simulink model "UAV_Task3"  (R2024b)
settings: Solver=VariableStepAuto  StartTime=0  StopTime=200  RelTol=1e-5  AbsTol=1e-5
values from neighbouring files (symbols this model uses):
  adaptiveActivation = 1    [Simplified_UAV_Task3_main.m]    (also in newUAV_Task3_main.m)
  B_p = 1/UAV.m    [Simplified_UAV_Task3_main.m]    (also in newUAV_Task3_main.m)
  F2plus = F2'*pinv(F2*F2')    [Simplified_UAV_Task3_main.m]    (also in newUAV_Task3_main.m)
  Gamma_a = 1*[1 1 1 1]'    [Simplified_UAV_Task3_main.m]    (also in newUAV_Task3_main.m = 2*[1 1 1 1]')
  gravityInAdaptiveController = 1    [Simplified_UAV_Task3_main.m]    (also in newUAV_Task3_main.m)
  k_f = 0.3379e-6    (= 3.379e-07)    [Simplified_UAV_Task3_main.m]    (also in newUAV_Task3_main.m)
  L = 10    [Simplified_UAV_Task3_main.m]    (also in newUAV_Task3_main.m)
  lambda_0 = 1    [Simplified_UAV_Task3_main.m]    (also in newUAV_Task3_main.m)
  Omega_0 = [1500 1500 1500 1500]'    [Simplified_UAV_Task3_main.m]    (also in newUAV_Task3_main.m)
  omegab_0 = [0; 0; 0]    [Simplified_UAV_Task3_main.m]    (also in newUAV_Task3_main.m)
  p_0 = [0; 0; 0]    [Simplified_UAV_Task3_main.m]    (also in newUAV_Task3_main.m)
  PO = 1    [Simplified_UAV_Task3_main.m]    (also in newUAV_Task3_main.m)
  q_0 = eul2quat([0, 0, 0]*degToRad,'ZYX')'    [Simplified_UAV_Task3_main.m]    (also in newUAV_Task3_main.m)
  scenario = 2    [Simplified_UAV_Task3_main.m]    (also in newUAV_Task3_main.m)
  theta_0 = [0.07;0.07;0.1]    [Simplified_UAV_Task3_main.m]    (also in newUAV_Task3_main.m)
  vb_0 = [0; 0; 0]    [Simplified_UAV_Task3_main.m]    (also in newUAV_Task3_main.m)
undefined symbols (not defined in the file or in its folder): adaptive_controller, ctrl, D_fv_i, dyn, e_3, epsilon_PO, fw_params_fc, g, Gamma_a_scalar, lambda_i, par, pos, pos_pp, projection_operator, targetParams, theta_M, UAV, v_M, vel, vel_pp
libraries: slpidlib x22, matrix_library x6, aerolibutil x2, uavutilslib x1
(part 2 of 4)

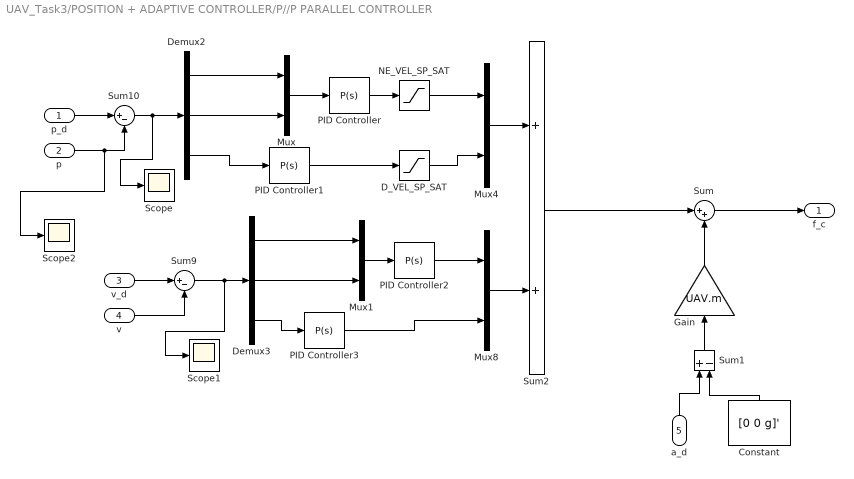
== system UAV_Task3/POSITION + ADAPTIVE CONTROLLER/P//P PARALLEL CONTROLLER ==
  p_d : Inport
  p : Inport  Port=2
  v_d : Inport  Port=3
  v : Inport  Port=4
  a_d : Inport  Port=5
  Constant : Constant  Value=[0 0 g]'
  D_VEL_SP_SAT : Saturate  UpperLimit=fw_params_fc.MPC_Z_VEL_MAX_DN  LowerLimit=-fw_params_fc.MPC_Z_VEL_MAX_UP
  Demux2 : Demux  Outputs=3
  Demux3 : Demux  Outputs=3
  Gain : Gain  Gain=UAV.m
  Mux{,1,4,8} (4 alike) : Mux  Inputs=2
  NE_VEL_SP_SAT : Saturate  UpperLimit=fw_params_fc.MPC_XY_VEL_MAX  LowerLimit=-fw_params_fc.MPC_XY_VEL_MAX
  PID Controller : slpidlib/PID Controller  Controller=P  Form=Parallel  TimeDomain=Continuous-time  UseExternalTs=off  SampleTime=-1  IntegratorMethod=Forward Euler  FilterMethod=Forward Euler  ControllerParametersSource=internal  P=pos_pp.Kp(1,1)  I=1  UseKiTs=off  D=0  UseExternalDerivativeSource=off  N=100  UseFilter=on  TunerSelectOption=Transfer Function Based (PID Tuner App)  InitialConditionSource=internal  InitialConditionForIntegrator=0  InitialConditionForFilter=0  DifferentiatorICPrevScaledInput=0  ExternalReset=none  TrackingMode=off  Kt=1  LimitOutput=off  SatLimitsSource=internal  UpperSaturationLimit=inf  LowerSaturationLimit=-inf  LinearizeAsGain=on  AntiWindupMode=none  Kb=1  LimitIntegrator=off  UpperIntegratorSaturationLimit=inf  LowerIntegratorSaturationLimit=-inf  POutMin=[]  POutMax=[]  IOutMin=[]  IOutMax=[]  DOutMin=[]  DOutMax=[]  NOutMin=[]  NOutMax=[]  SumOutMin=[]  SumOutMax=[]  SaturationOutMin=[]  SaturationOutMax=[]  PParamMin=[]  PParamMax=[]  IParamMin=[]  IParamMax=[]  DParamMin=[]  DParamMax=[]  NParamMin=[]  NParamMax=[]  KbParamMin=[]  KbParamMax=[]  KtParamMin=[]  KtParamMax=[]  KbOutMin=[]  KbOutMax=[]  KtOutMin=[]  KtOutMax=[]  IntegratorOutMin=[]  IntegratorOutMax=[]  FilterOutMin=[]  FilterOutMax=[]  SumI1OutMin=[]  SumI1OutMax=[]  SumI2OutMin=[]  SumI2OutMax=[]  SumI3OutMin=[]  SumI3OutMax=[]  SumI4OutMin=[]  SumI4OutMax=[]  SumDOutMin=[]  SumDOutMax=[]  DifferentiatorOutMin=[]  DifferentiatorOutMax=[]  FilterDiffOutCoefMin=[]  FilterDiffOutCoefMax=[]  ReciprocalOutMin=[]  ReciprocalOutMax=[]  SumDenOutMin=[]  SumDenOutMax=[]  SumNumOutMin=[]  SumNumOutMax=[]  DivideOutMin=[]  DivideOutMax=[]  UdiffTsProdOutMin=[]  UdiffTsProdOutMax=[]  NTsProdOutMin=[]  NTsProdOutMax=[]  UintegralTsProdOutMin=[]  UintegralTsProdOutMax=[]  UngainTsProdOutMin=[]  UngainTsProdOutMax=[]  ClampingZeroOutDataTypeStr=Inherit: Inherit via back propagation  ClampingZeroOutMin=[]  ClampingZeroOutMax=[]  FilterDenConstantOutDataTypeStr=Inherit: Inherit via back propagation  FilterDenConstantOutMin=[]  FilterDenConstantOutMax=[]  PCopyOutDataTypeStr=Inherit: Inherit via back propagation  PCopyOutMin=[]  PCopyOutMax=[]  NCopyOutDataTypeStr=Inherit: Inherit via back propagation  NCopyOutMin=[]  NCopyOutMax=[]  IntegratorContinuousStateAttributes=''  IntegratorStateMustResolveToSignalObject=off  IntegratorRTWStateStorageClass=Auto  FilterContinuousStateAttributes=''  FilterStateMustResolveToSignalObject=off  FilterRTWStateStorageClass=Auto  ParallelPVariant=InternalParameters  IdealPVariant=Disabled  IVariant=Disabled  DVariant=Disabled  IntegratorVariant=Disabled  SatVariant=Disabled  AWVariant=Disabled  PCopyVariant=Disabled  TRVariant=Disabled  FdbkBlocksVariant=Forward  IdealPFdbkVariant=Disabled  SatFdbkVariant=Disabled  DerivativeFilterVariant=Disabled  NVariant=Disabled  NCopyVariant=Disabled_SignalSpec  FilterICVariant=Disabled  IntegratorICVariant=Disabled  ExternalResetVariant=Disabled  TRSumVariant=Passthrough  SumFdbkVariant=Disabled  SumVariant=Passthrough_P  TsampFilterVariant=InternalTs  TsampNgainVariant=Passthrough  TsampIntegralVariant=Disabled_SignalSpec  ExternalSaturationOutDataTypeStr=Inherit: Same as second input  DerivativeSourceVariant=Disabled  PreIntVariant=InternalPreInt
  PID Controller1 : slpidlib/PID Controller  Controller=P  Form=Parallel  TimeDomain=Continuous-time  UseExternalTs=off  SampleTime=-1  IntegratorMethod=Forward Euler  FilterMethod=Forward Euler  ControllerParametersSource=internal  P=pos_pp.Kp(3,3)  I=6.65250446585681  UseKiTs=off  D=9.35493624576525  UseExternalDerivativeSource=off  N=3445.77467620609  UseFilter=on  TunerSelectOption=Transfer Function Based (PID Tuner App)  InitialConditionSource=internal  InitialConditionForIntegrator=0  InitialConditionForFilter=0  DifferentiatorICPrevScaledInput=0  ExternalReset=none  TrackingMode=off  Kt=1  LimitOutput=off  SatLimitsSource=internal  UpperSaturationLimit=inf  LowerSaturationLimit=-inf  LinearizeAsGain=on  AntiWindupMode=none  Kb=1  LimitIntegrator=off  UpperIntegratorSaturationLimit=inf  LowerIntegratorSaturationLimit=-inf  POutMin=[]  POutMax=[]  IOutMin=[]  IOutMax=[]  DOutMin=[]  DOutMax=[]  NOutMin=[]  NOutMax=[]  SumOutMin=[]  SumOutMax=[]  SaturationOutMin=[]  SaturationOutMax=[]  PParamMin=[]  PParamMax=[]  IParamMin=[]  IParamMax=[]  DParamMin=[]  DParamMax=[]  NParamMin=[]  NParamMax=[]  KbParamMin=[]  KbParamMax=[]  KtParamMin=[]  KtParamMax=[]  KbOutMin=[]  KbOutMax=[]  KtOutMin=[]  KtOutMax=[]  IntegratorOutMin=[]  IntegratorOutMax=[]  FilterOutMin=[]  FilterOutMax=[]  SumI1OutMin=[]  SumI1OutMax=[]  SumI2OutMin=[]  SumI2OutMax=[]  SumI3OutMin=[]  SumI3OutMax=[]  SumI4OutMin=[]  SumI4OutMax=[]  SumDOutMin=[]  SumDOutMax=[]  DifferentiatorOutMin=[]  DifferentiatorOutMax=[]  FilterDiffOutCoefMin=[]  FilterDiffOutCoefMax=[]  ReciprocalOutMin=[]  ReciprocalOutMax=[]  SumDenOutMin=[]  SumDenOutMax=[]  SumNumOutMin=[]  SumNumOutMax=[]  DivideOutMin=[]  DivideOutMax=[]  UdiffTsProdOutMin=[]  UdiffTsProdOutMax=[]  NTsProdOutMin=[]  NTsProdOutMax=[]  UintegralTsProdOutMin=[]  UintegralTsProdOutMax=[]  UngainTsProdOutMin=[]  UngainTsProdOutMax=[]  ClampingZeroOutDataTypeStr=Inherit: Inherit via back propagation  ClampingZeroOutMin=[]  ClampingZeroOutMax=[]  FilterDenConstantOutDataTypeStr=Inherit: Inherit via back propagation  FilterDenConstantOutMin=[]  FilterDenConstantOutMax=[]  PCopyOutDataTypeStr=Inherit: Inherit via back propagation  PCopyOutMin=[]  PCopyOutMax=[]  NCopyOutDataTypeStr=Inherit: Inherit via back propagation  NCopyOutMin=[]  NCopyOutMax=[]  IntegratorContinuousStateAttributes=''  IntegratorStateMustResolveToSignalObject=off  IntegratorRTWStateStorageClass=Auto  FilterContinuousStateAttributes=''  FilterStateMustResolveToSignalObject=off  FilterRTWStateStorageClass=Auto  ParallelPVariant=InternalParameters  IdealPVariant=Disabled  IVariant=Disabled  DVariant=Disabled  IntegratorVariant=Disabled  SatVariant=Disabled  AWVariant=Disabled  PCopyVariant=Disabled  TRVariant=Disabled  FdbkBlocksVariant=Forward  IdealPFdbkVariant=Disabled  SatFdbkVariant=Disabled  DerivativeFilterVariant=Disabled  NVariant=Disabled  NCopyVariant=Disabled_SignalSpec  FilterICVariant=Disabled  IntegratorICVariant=Disabled  ExternalResetVariant=Disabled  TRSumVariant=Passthrough  SumFdbkVariant=Disabled  SumVariant=Passthrough_P  TsampFilterVariant=InternalTs  TsampNgainVariant=Passthrough  TsampIntegralVariant=Disabled_SignalSpec  ExternalSaturationOutDataTypeStr=Inherit: Same as second input  DerivativeSourceVariant=Disabled  PreIntVariant=InternalPreInt
  PID Controller2 : slpidlib/PID Controller  Controller=P  Form=Parallel  TimeDomain=Continuous-time  UseExternalTs=off  SampleTime=-1  IntegratorMethod=Forward Euler  FilterMethod=Forward Euler  ControllerParametersSource=internal  P=vel_pp.Kp(1,1)  I=1  UseKiTs=off  D=0  UseExternalDerivativeSource=off  N=100  UseFilter=on  TunerSelectOption=Transfer Function Based (PID Tuner App)  InitialConditionSource=internal  InitialConditionForIntegrator=0  InitialConditionForFilter=0  DifferentiatorICPrevScaledInput=0  ExternalReset=none  TrackingMode=off  Kt=1  LimitOutput=off  SatLimitsSource=internal  UpperSaturationLimit=inf  LowerSaturationLimit=-inf  LinearizeAsGain=on  AntiWindupMode=none  Kb=1  LimitIntegrator=off  UpperIntegratorSaturationLimit=inf  LowerIntegratorSaturationLimit=-inf  POutMin=[]  POutMax=[]  IOutMin=[]  IOutMax=[]  DOutMin=[]  DOutMax=[]  NOutMin=[]  NOutMax=[]  SumOutMin=[]  SumOutMax=[]  SaturationOutMin=[]  SaturationOutMax=[]  PParamMin=[]  PParamMax=[]  IParamMin=[]  IParamMax=[]  DParamMin=[]  DParamMax=[]  NParamMin=[]  NParamMax=[]  KbParamMin=[]  KbParamMax=[]  KtParamMin=[]  KtParamMax=[]  KbOutMin=[]  KbOutMax=[]  KtOutMin=[]  KtOutMax=[]  IntegratorOutMin=[]  IntegratorOutMax=[]  FilterOutMin=[]  FilterOutMax=[]  SumI1OutMin=[]  SumI1OutMax=[]  SumI2OutMin=[]  SumI2OutMax=[]  SumI3OutMin=[]  SumI3OutMax=[]  SumI4OutMin=[]  SumI4OutMax=[]  SumDOutMin=[]  SumDOutMax=[]  DifferentiatorOutMin=[]  DifferentiatorOutMax=[]  FilterDiffOutCoefMin=[]  FilterDiffOutCoefMax=[]  ReciprocalOutMin=[]  ReciprocalOutMax=[]  SumDenOutMin=[]  SumDenOutMax=[]  SumNumOutMin=[]  SumNumOutMax=[]  DivideOutMin=[]  DivideOutMax=[]  UdiffTsProdOutMin=[]  UdiffTsProdOutMax=[]  NTsProdOutMin=[]  NTsProdOutMax=[]  UintegralTsProdOutMin=[]  UintegralTsProdOutMax=[]  UngainTsProdOutMin=[]  UngainTsProdOutMax=[]  ClampingZeroOutDataTypeStr=Inherit: Inherit via back propagation  ClampingZeroOutMin=[]  ClampingZeroOutMax=[]  FilterDenConstantOutDataTypeStr=Inherit: Inherit via back propagation  FilterDenConstantOutMin=[]  FilterDenConstantOutMax=[]  PCopyOutDataTypeStr=Inherit: Inherit via back propagation  PCopyOutMin=[]  PCopyOutMax=[]  NCopyOutDataTypeStr=Inherit: Inherit via back propagation  NCopyOutMin=[]  NCopyOutMax=[]  IntegratorContinuousStateAttributes=''  IntegratorStateMustResolveToSignalObject=off  IntegratorRTWStateStorageClass=Auto  FilterContinuousStateAttributes=''  FilterStateMustResolveToSignalObject=off  FilterRTWStateStorageClass=Auto  ParallelPVariant=InternalParameters  IdealPVariant=Disabled  IVariant=Disabled  DVariant=Disabled  IntegratorVariant=Disabled  SatVariant=Disabled  AWVariant=Disabled  PCopyVariant=Disabled  TRVariant=Disabled  FdbkBlocksVariant=Forward  IdealPFdbkVariant=Disabled  SatFdbkVariant=Disabled  DerivativeFilterVariant=Disabled  NVariant=Disabled  NCopyVariant=Disabled_SignalSpec  FilterICVariant=Disabled  IntegratorICVariant=Disabled  ExternalResetVariant=Disabled  TRSumVariant=Passthrough  SumFdbkVariant=Disabled  SumVariant=Passthrough_P  TsampFilterVariant=InternalTs  TsampNgainVariant=Passthrough  TsampIntegralVariant=Disabled_SignalSpec  ExternalSaturationOutDataTypeStr=Inherit: Same as second input  DerivativeSourceVariant=Disabled  PreIntVariant=InternalPreInt
  PID Controller3 : slpidlib/PID Controller  Controller=P  Form=Parallel  TimeDomain=Continuous-time  UseExternalTs=off  SampleTime=-1  IntegratorMethod=Forward Euler  FilterMethod=Forward Euler  ControllerParametersSource=internal  P=vel_pp.Kp(3,3)  I=1  UseKiTs=off  D=0  UseExternalDerivativeSource=off  N=100  UseFilter=on  TunerSelectOption=Transfer Function Based (PID Tuner App)  InitialConditionSource=internal  InitialConditionForIntegrator=0  InitialConditionForFilter=0  DifferentiatorICPrevScaledInput=0  ExternalReset=none  TrackingMode=off  Kt=1  LimitOutput=off  SatLimitsSource=internal  UpperSaturationLimit=inf  LowerSaturationLimit=-inf  LinearizeAsGain=on  AntiWindupMode=none  Kb=1  LimitIntegrator=off  UpperIntegratorSaturationLimit=inf  LowerIntegratorSaturationLimit=-inf  POutMin=[]  POutMax=[]  IOutMin=[]  IOutMax=[]  DOutMin=[]  DOutMax=[]  NOutMin=[]  NOutMax=[]  SumOutMin=[]  SumOutMax=[]  SaturationOutMin=[]  SaturationOutMax=[]  PParamMin=[]  PParamMax=[]  IParamMin=[]  IParamMax=[]  DParamMin=[]  DParamMax=[]  NParamMin=[]  NParamMax=[]  KbParamMin=[]  KbParamMax=[]  KtParamMin=[]  KtParamMax=[]  KbOutMin=[]  KbOutMax=[]  KtOutMin=[]  KtOutMax=[]  IntegratorOutMin=[]  IntegratorOutMax=[]  FilterOutMin=[]  FilterOutMax=[]  SumI1OutMin=[]  SumI1OutMax=[]  SumI2OutMin=[]  SumI2OutMax=[]  SumI3OutMin=[]  SumI3OutMax=[]  SumI4OutMin=[]  SumI4OutMax=[]  SumDOutMin=[]  SumDOutMax=[]  DifferentiatorOutMin=[]  DifferentiatorOutMax=[]  FilterDiffOutCoefMin=[]  FilterDiffOutCoefMax=[]  ReciprocalOutMin=[]  ReciprocalOutMax=[]  SumDenOutMin=[]  SumDenOutMax=[]  SumNumOutMin=[]  SumNumOutMax=[]  DivideOutMin=[]  DivideOutMax=[]  UdiffTsProdOutMin=[]  UdiffTsProdOutMax=[]  NTsProdOutMin=[]  NTsProdOutMax=[]  UintegralTsProdOutMin=[]  UintegralTsProdOutMax=[]  UngainTsProdOutMin=[]  UngainTsProdOutMax=[]  ClampingZeroOutDataTypeStr=Inherit: Inherit via back propagation  ClampingZeroOutMin=[]  ClampingZeroOutMax=[]  FilterDenConstantOutDataTypeStr=Inherit: Inherit via back propagation  FilterDenConstantOutMin=[]  FilterDenConstantOutMax=[]  PCopyOutDataTypeStr=Inherit: Inherit via back propagation  PCopyOutMin=[]  PCopyOutMax=[]  NCopyOutDataTypeStr=Inherit: Inherit via back propagation  NCopyOutMin=[]  NCopyOutMax=[]  IntegratorContinuousStateAttributes=''  IntegratorStateMustResolveToSignalObject=off  IntegratorRTWStateStorageClass=Auto  FilterContinuousStateAttributes=''  FilterStateMustResolveToSignalObject=off  FilterRTWStateStorageClass=Auto  ParallelPVariant=InternalParameters  IdealPVariant=Disabled  IVariant=Disabled  DVariant=Disabled  IntegratorVariant=Disabled  SatVariant=Disabled  AWVariant=Disabled  PCopyVariant=Disabled  TRVariant=Disabled  FdbkBlocksVariant=Forward  IdealPFdbkVariant=Disabled  SatFdbkVariant=Disabled  DerivativeFilterVariant=Disabled  NVariant=Disabled  NCopyVariant=Disabled_SignalSpec  FilterICVariant=Disabled  IntegratorICVariant=Disabled  ExternalResetVariant=Disabled  TRSumVariant=Passthrough  SumFdbkVariant=Disabled  SumVariant=Passthrough_P  TsampFilterVariant=InternalTs  TsampNgainVariant=Passthrough  TsampIntegralVariant=Disabled_SignalSpec  ExternalSaturationOutDataTypeStr=Inherit: Same as second input  DerivativeSourceVariant=Disabled  PreIntVariant=InternalPreInt
  Scope : Scope
  Scope1 : Scope
  Scope2 : Scope
  Sum : Sum  Inputs=|++
  Sum1 : Sum  Inputs=+-
  Sum10 : Sum  Inputs=|+-
  Sum2 : Sum
  Sum9 : Sum  Inputs=|+-
  f_c : Outport
  wires:
  p_d/1 -> Sum10/1
  p/1 -> Scope2/1, Sum10/2
  v_d/1 -> Sum9/1
  Sum9/1 -> Scope1/1, Demux3/1
  Sum10/1 -> Scope/1, Demux2/1
  Demux3/3 -> PID Controller3/1
  v/1 -> Sum9/2
  Demux2/3 -> PID Controller1/1
  Mux4/1 -> Sum2/1
  Mux8/1 -> Sum2/2
  Demux2/2 -> Mux/2
  Sum/1 -> f_c/1
  Gain/1 -> Sum/2
  Sum1/1 -> Gain/1
  a_d/1 -> Sum1/1
  Constant/1 -> Sum1/2
  Sum2/1 -> Sum/1
  Mux/1 -> PID Controller/1
  Demux2/1 -> Mux/1
  Demux3/1 -> Mux1/1
  Demux3/2 -> Mux1/2
  Mux1/1 -> PID Controller2/1
  PID Controller3/1 -> Mux8/2
  PID Controller2/1 -> Mux8/1
  PID Controller/1 -> NE_VEL_SP_SAT/1
  NE_VEL_SP_SAT/1 -> Mux4/1
  PID Controller1/1 -> D_VEL_SP_SAT/1
  D_VEL_SP_SAT/1 -> Mux4/2

== system UAV_Task3/POSITION + ADAPTIVE CONTROLLER/POSITION CONTROLLER ==
  p_d : Inport
  p : Inport  Port=2
  v_d : Inport  Port=3
  v : Inport  Port=4
  a_d : Inport  Port=5
  Position controller : Subsystem
  Scope : Scope
  Sum : Sum  Inputs=|+-
  Velocity Controller : Subsystem
  f_c : Outport
  wires:
  v/1 -> Position controller/5(v), Velocity Controller/1(v)
  Position controller/1(" v_c") -> Velocity Controller/2(v_c)
  Position controller/2(" a_c") -> Velocity Controller/3(a_c)
  a_d/1 -> Position controller/4(a_d)
  v_d/1 -> Position controller/3(v_d)
  p/1 -> Sum/1, Position controller/1(p)
  p_d/1 -> Sum/2, Position controller/2(p_d)
  Sum/1 -> Scope/1
  Velocity Controller/1(f_c) -> f_c/1

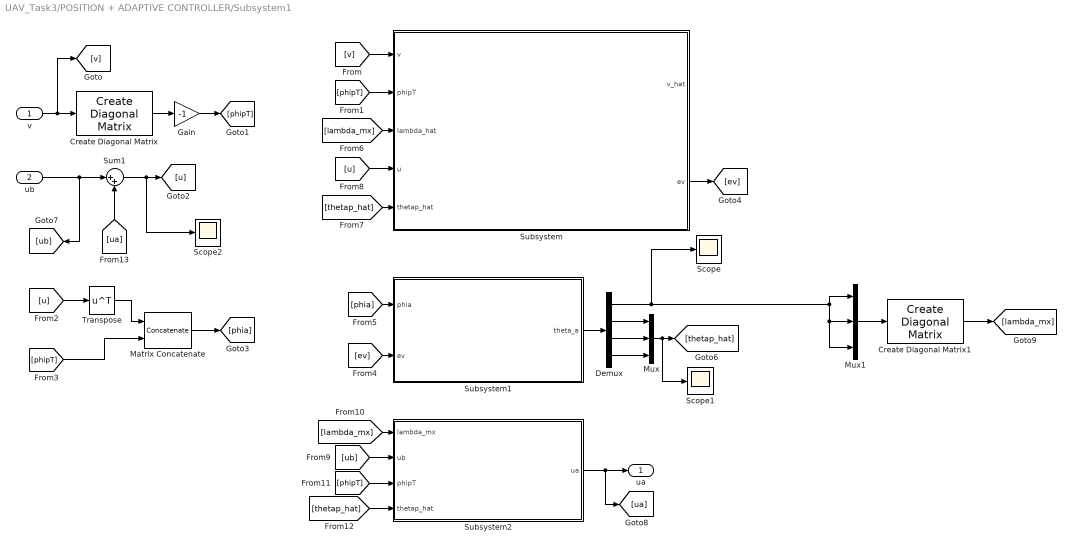
== system UAV_Task3/POSITION + ADAPTIVE CONTROLLER/Subsystem1 ==
  v : Inport
  ub : Inport  Port=2
  Create Diagonal Matrix : matrix_library/Create Diagonal Matrix
  Create Diagonal Matrix1 : matrix_library/Create Diagonal Matrix
  Demux : Demux
  Gain : Gain  Gain=-1
  Matrix Concatenate : Concatenate  Mode=Multidimensional array
  Mux : Mux  Inputs=3
  Mux1 : Mux  Inputs=3
  Scope : Scope
  Scope1 : Scope
  Scope2 : Scope
  Subsystem : Subsystem
  Subsystem1 : Subsystem
  Subsystem2 : Subsystem
  Sum1 : Sum  Inputs=|++
  Transpose : Math  Operator=transpose
  ua : Outport
  wires:
  v/1 -> [v], Create Diagonal Matrix/1
  ub/1 -> Sum1/1, [ub]
  [v] -> Subsystem/1(v)
  [phipT] -> Subsystem/2(phipT)
  [phipT] -> Matrix Concatenate/2
  Subsystem/2(ev) -> [ev]
  [ev] -> Subsystem1/2(ev)
  [phia] -> Subsystem1/1(phia)
  Subsystem1/1(theta_a) -> Demux/1
  Demux/4 -> Mux/3
  Demux/3 -> Mux/2
  Demux/2 -> Mux/1
  Mux/1 -> Scope1/1, [thetap_hat]
  [lambda_mx] -> Subsystem/3(lambda_hat)
  [thetap_hat] -> Subsystem/5(thetap_hat)
  [u] -> Subsystem/4(u)
  [ub] -> Subsystem2/2(ub)
  [phipT] -> Subsystem2/3(phipT)
  [thetap_hat] -> Subsystem2/4(thetap_hat)
  Subsystem2/1(ua) -> [ua], ua/1
  [ua] -> Sum1/2
  Demux/1 -> Scope/1, Mux1/1, Mux1/3, Mux1/2
  Mux1/1 -> Create Diagonal Matrix1/1
  Create Diagonal Matrix1/1 -> [lambda_mx]
  [lambda_mx] -> Subsystem2/1(lambda_mx)
  Create Diagonal Matrix/1 -> Gain/1
  Gain/1 -> [phipT]
  [u] -> Transpose/1
  Matrix Concatenate/1 -> [phia]
  Sum1/1 -> Scope2/1, [u]
  Transpose/1 -> Matrix Concatenate/1

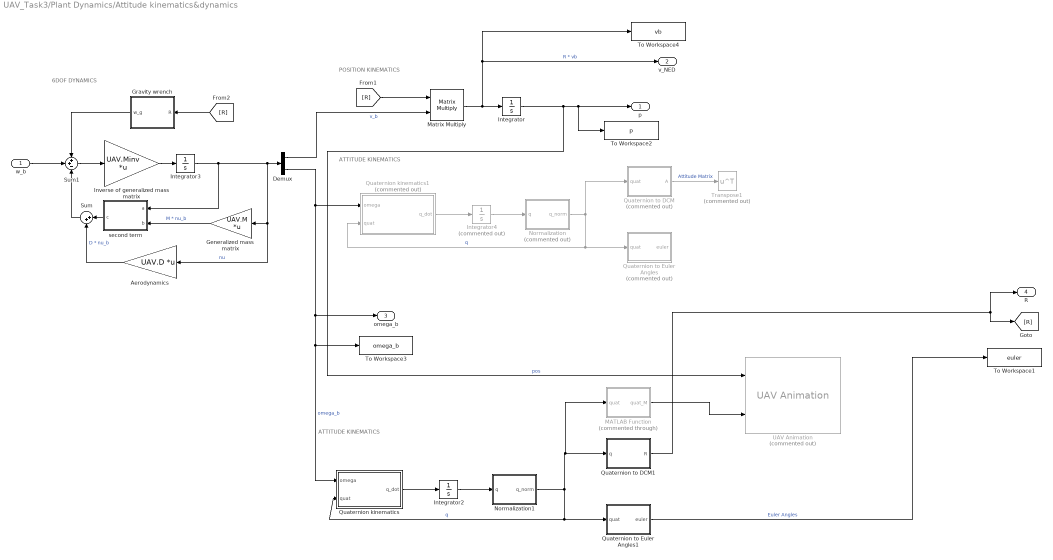
== system UAV_Task3/Plant Dynamics/Attitude kinematics&dynamics ==
  note: POSITION KINEMATICS
  note: ATTITUDE KINEMATICS
  note: 6DOF DYNAMICS
  note: ATTITUDE KINEMATICS
  w_b : Inport
  Aerodynamics : Gain  Gain=UAV.D  Multiplication=Matrix(K*u)
  Demux : Demux  Outputs=2
  Generalized mass matrix : Gain  Gain=UAV.M  Multiplication=Matrix(K*u)
  Gravity wrench : MATLAB Function  TreatAsAtomicUnit=on
  Integrator : Integrator  InitialCondition=p_0
  Integrator2 : Integrator  InitialCondition=q_0
  Integrator3 : Integrator  InitialCondition=[vb_0;omegab_0]
  Integrator4 : Integrator  Commented=on  InitialCondition=q_0
  Inverse of generalized mass matrix : Gain  Gain=UAV.Minv  Multiplication=Matrix(K*u)
  MATLAB Function : MATLAB Function  Commented=through  TreatAsAtomicUnit=on
  Matrix Multiply : Product  Multiplication=Matrix(*)
  Normalization : MATLAB Function  Commented=on  TreatAsAtomicUnit=on
  Normalization1 : MATLAB Function  TreatAsAtomicUnit=on
  Quaternion kinematics : MATLAB Function  TreatAsAtomicUnit=on
  Quaternion kinematics1 : MATLAB Function  Commented=on  TreatAsAtomicUnit=on
  Quaternion to DCM : MATLAB Function  Commented=on  TreatAsAtomicUnit=on
  Quaternion to DCM1 : MATLAB Function  TreatAsAtomicUnit=on
  Quaternion to Euler Angles : MATLAB Function  Commented=on  TreatAsAtomicUnit=on
  Quaternion to Euler Angles1 : MATLAB Function  TreatAsAtomicUnit=on
  Sum : Sum  Inputs=|++
  Sum1 : Sum  Inputs=++-
  To Workspace1 : ToWorkspace  VariableName=euler  SaveFormat=Timeseries  SampleTime=-1
  To Workspace2 : ToWorkspace  VariableName=p  SaveFormat=Timeseries  SampleTime=-1
  To Workspace3 : ToWorkspace  VariableName=omega_b  SaveFormat=Timeseries  SampleTime=-1
  To Workspace4 : ToWorkspace  VariableName=vb  SaveFormat=Timeseries  SampleTime=-1
  Transpose1 : Math  Commented=on  Operator=transpose
  UAV Animation : uavutilslib/UAV Animation  Commented=on  NumUAV=1  DynamicUAVConfig=off  UAVType=Multirotor  UAVSize=1  UAVColor=[1 0 0]  UAVTrajectoryAlpha=1  InertialZDirection=Down  RotationFormat=Quaternion  DrawMarkers=off  SampleTime=-1
  "second term " : MATLAB Function  TreatAsAtomicUnit=on
  p : Outport
  v_NED : Outport  Port=2
  omega_b : Outport  Port=3
  R : Outport  Port=4
  wires:
  Matrix Multiply/1 -> v_NED/1, To Workspace4/1, Integrator/1  "R * vb"
  Integrator/1 -> UAV Animation/1, p/1, To Workspace2/1  "pos"
  Sum1/1 -> Inverse of generalized mass matrix/1
  Quaternion kinematics1/1(q_dot) -> Integrator4/1
  Generalized mass matrix/1 -> "second term "/2(b)  "M * nu_b"
  Demux/1 -> Matrix Multiply/2  "v_b"
  Quaternion to Euler Angles1/1(euler) -> To Workspace1/1  "Euler Angles"
  Inverse of generalized mass matrix/1 -> Integrator3/1
  Integrator4/1 -> Normalization/1(q)
  Quaternion to DCM/1(A) -> Transpose1/1  "Attitude Matrix"
  Integrator3/1 -> Aerodynamics/1, Generalized mass matrix/1, Demux/1, "second term "/1(a)  "nu"
  [R] -> Matrix Multiply/1
  [R] -> Gravity wrench/1(R)
  w_b/1 -> Sum1/2
  Gravity wrench/1(w_g) -> Sum1/1
  Normalization/1(q_norm) -> Quaternion kinematics1/2(quat), Quaternion to Euler Angles/1(quat), Quaternion to DCM/1(quat)  "q"
  Quaternion kinematics/1(q_dot) -> Integrator2/1
  Integrator2/1 -> Normalization1/1(q)
  Normalization1/1(q_norm) -> Quaternion kinematics/2(quat), Quaternion to Euler Angles1/1(quat), MATLAB Function/1(quat), Quaternion to DCM1/1(q)  "q"
  Demux/2 -> omega_b/1, Quaternion kinematics/1(omega), To Workspace3/1, Quaternion kinematics1/1(omega)  "omega_b"
  Quaternion to DCM1/1(R) -> R/1, [R]
  MATLAB Function/1(quat_M) -> UAV Animation/2
  "second term "/1(c) -> Sum/1
  Sum/1 -> Sum1/3
  Aerodynamics/1 -> Sum/2  "D * nu_b"

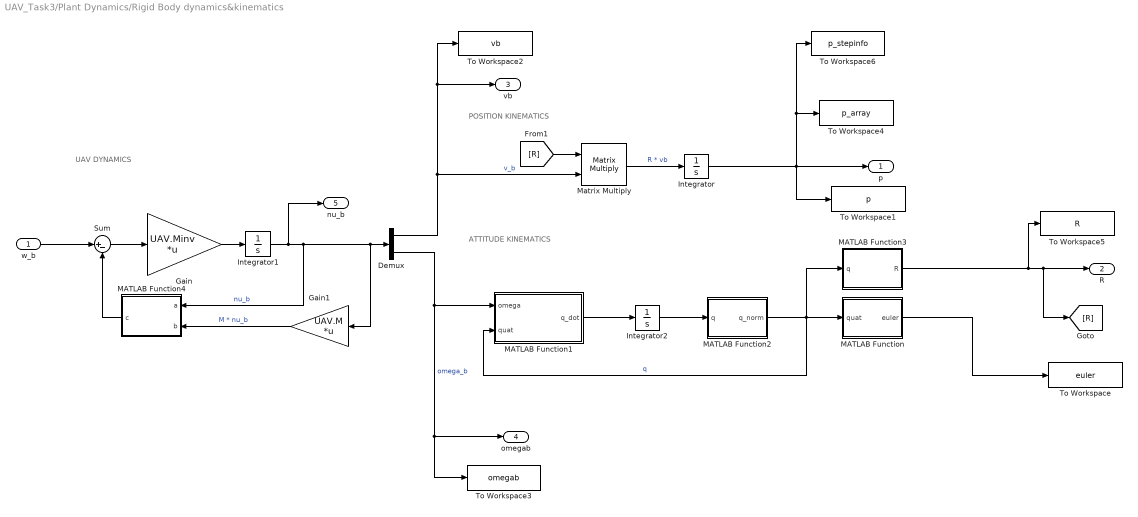
== system UAV_Task3/Plant Dynamics/Rigid Body dynamics&kinematics  ==
  note: UAV DYNAMICS
  note: ATTITUDE KINEMATICS
  note: POSITION KINEMATICS
  w_b : Inport
  Demux : Demux  Outputs=2
  Gain : Gain  Gain=UAV.Minv  Multiplication=Matrix(K*u)
  Gain1 : Gain  Gain=UAV.M  Multiplication=Matrix(K*u)
  Integrator : Integrator  InitialCondition=p_0
  Integrator1 : Integrator  InitialCondition=[vb_0;omegab_0]
  Integrator2 : Integrator  InitialCondition=q_0
  MATLAB Function : MATLAB Function  TreatAsAtomicUnit=on
  MATLAB Function1 : MATLAB Function  TreatAsAtomicUnit=on
  MATLAB Function2 : MATLAB Function  TreatAsAtomicUnit=on
  MATLAB Function3 : MATLAB Function  TreatAsAtomicUnit=on
  MATLAB Function4 : MATLAB Function  TreatAsAtomicUnit=on
  Matrix Multiply : Product  Multiplication=Matrix(*)
  Sum : Sum  Inputs=|+-
  To Workspace : ToWorkspace  VariableName=euler  SaveFormat=Timeseries  SampleTime=-1
  To Workspace1 : ToWorkspace  VariableName=p  SaveFormat=Timeseries  SampleTime=-1
  To Workspace2 : ToWorkspace  VariableName=vb  SaveFormat=Timeseries  SampleTime=-1
  To Workspace3 : ToWorkspace  VariableName=omegab  SaveFormat=Timeseries  SampleTime=-1
  To Workspace4 : ToWorkspace  VariableName=p_array  SampleTime=-1
  To Workspace5 : ToWorkspace  VariableName=R  SaveFormat=Structure With Time  SampleTime=-1
  To Workspace6 : ToWorkspace  VariableName=p_stepinfo  SaveFormat=Structure With Time  SampleTime=-1
  p : Outport
  R : Outport  Port=2
  vb : Outport  Port=3
  omegab : Outport  Port=4
  nu_b : Outport  Port=5
  wires:
  Integrator/1 -> To Workspace6/1, To Workspace4/1, p/1, To Workspace1/1
  MATLAB Function1/1(q_dot) -> Integrator2/1
  MATLAB Function2/1(q_norm) -> MATLAB Function3/1(q), MATLAB Function1/2(quat), MATLAB Function/1(quat)  "q"
  MATLAB Function3/1(R) -> R/1, [R], To Workspace5/1
  Demux/1 -> vb/1, To Workspace2/1, Matrix Multiply/2  "v_b"
  Integrator1/1 -> nu_b/1, Demux/1, Gain1/1, MATLAB Function4/1(a)  "nu_b"
  Integrator2/1 -> MATLAB Function2/1(q)
  Matrix Multiply/1 -> Integrator/1  "R * vb"
  MATLAB Function/1(euler) -> To Workspace/1
  [R] -> Matrix Multiply/1
  Gain/1 -> Integrator1/1
  Demux/2 -> omegab/1, To Workspace3/1, MATLAB Function1/1(omega)  "omega_b"
  Gain1/1 -> MATLAB Function4/2(b)  "M * nu_b"
  Sum/1 -> Gain/1
  MATLAB Function4/1(c) -> Sum/2
  w_b/1 -> Sum/1

== system UAV_Task3/Plant Dynamics/Rotor Dynamics ==
  T_cmd : Inport
  Gain : Gain  Gain=1/k_f
  Gain1 : Gain  Gain=sqrt(UAV.lambda_r)
  Gain2 : Gain  Gain=UAV.k_m
  Gain3 : Gain  Gain=k_f
  Integrator : Integrator  InitialCondition=Omega_0
  Saturation : Saturate  UpperLimit=UAV.T_max  LowerLimit=UAV.T_min
  Sqrt : Sqrt
  Square : Math  Operator=square
  Sum : Sum  Inputs=|+-
  Actual Thrust : Outport
  wires:
  Gain3/1 -> Saturation/1
  Integrator/1 -> Sum/2, Square/1  "Omega"
  Square/1 -> Gain3/1
  Gain/1 -> Sqrt/1
  Sqrt/1 -> Gain1/1  "Omega_cmd"
  Sum/1 -> Gain2/1
  Gain1/1 -> Sum/1
  Saturation/1 -> Actual Thrust/1  "Actual Thrust"
  T_cmd/1 -> Gain/1
  Gain2/1 -> Integrator/1

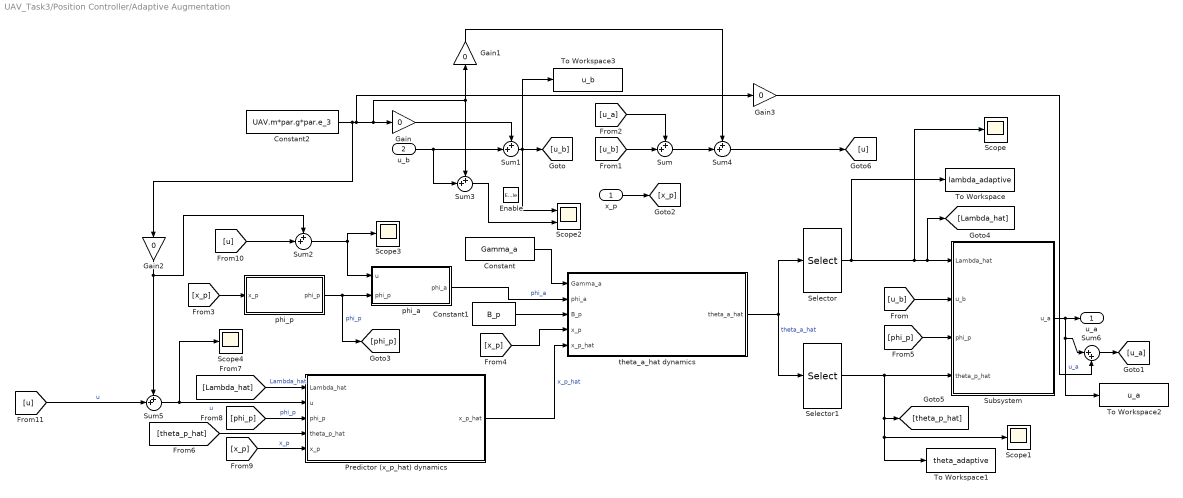
== system UAV_Task3/Position Controller/Adaptive Augmentation ==
  x_p : Inport
  u_b : Inport  Port=2
  Enable : EnablePort
  Constant : Constant  Value=Gamma_a
  Constant1 : Constant  Value=B_p
  Constant2 : Constant  Value=UAV.m*par.g*par.e_3
  Gain{,1..3} (4 alike) : Gain  Gain=0
  Predictor (x_p_hat) dynamics : Subsystem
  Scope{,1,3..4} (4 alike) : Scope
  Scope2 : Scope  NumInputPorts=2
  Selector : Selector  InputPortWidth=4  IndexOptions=Index vector (dialog)  Indices=[1]  OutputSizes=1
  Selector1 : Selector  InputPortWidth=4  IndexOptions=Index vector (dialog)  Indices=[2 3 4]  OutputSizes=1
  Subsystem : Subsystem
  Sum{,1..5} (6 alike) : Sum  Inputs=++|
  Sum6 : Sum  Inputs=|++
  To Workspace : ToWorkspace  VariableName=lambda_adaptive  SaveFormat=Timeseries  SampleTime=-1
  To Workspace1 : ToWorkspace  VariableName=theta_adaptive  SaveFormat=Timeseries  SampleTime=-1
  To Workspace2 : ToWorkspace  VariableName=u_a  SaveFormat=Timeseries  SampleTime=-1
  To Workspace3 : ToWorkspace  VariableName=u_b  SaveFormat=Timeseries  SampleTime=-1
  phi_a : Subsystem
  phi_p : Subsystem
  theta_a_hat dynamics : Subsystem
  u_a : Outport
  wires:
  Selector1/1 -> Subsystem/4(theta_p_hat), Scope1/1, To Workspace1/1, [theta_p_hat]
  theta_a_hat dynamics/1(theta_a_hat) -> Selector/1, Selector1/1  "theta_a_hat"
  Constant/1 -> theta_a_hat dynamics/1(Gamma_a)
  phi_p/1(phi_p) -> phi_a/2(phi_p), [phi_p]  "phi_p"
  [u_b] -> Sum/2
  phi_a/1(phi_a) -> theta_a_hat dynamics/2(phi_a)  "phi_a"
  [x_p] -> phi_p/1(x_p)
  [x_p] -> theta_a_hat dynamics/4(x_p)
  Constant1/1 -> theta_a_hat dynamics/3(B_p)
  [phi_p] -> Subsystem/3(phi_p)
  Predictor (x_p_hat) dynamics/1(x_p_hat) -> theta_a_hat dynamics/5(x_p_hat)  "x_p_hat"
  [theta_p_hat] -> Predictor (x_p_hat) dynamics/4(theta_p_hat)
  [Lambda_hat] -> Predictor (x_p_hat) dynamics/1(Lambda_hat)  "Lambda_hat"
  [phi_p] -> Predictor (x_p_hat) dynamics/3(phi_p)  "phi_p"
  [x_p] -> Predictor (x_p_hat) dynamics/5(x_p)  "x_p"
  x_p/1 -> [x_p]
  [u_a] -> Sum/1
  Selector/1 -> Scope/1, [Lambda_hat], Subsystem/1(Lambda_hat), To Workspace/1
  u_b/1 -> Sum3/2, Sum1/2
  Sum1/1 -> Scope2/1, To Workspace3/1, [u_b]
  [u_b] -> Subsystem/2(u_b)
  Subsystem/1(u_a) -> Sum6/1, To Workspace2/1, u_a/1  "u_a"
  Sum2/1 -> phi_a/1(u), Scope3/1
  [u] -> Sum2/2
  Gain/1 -> Sum1/1
  Sum3/1 -> Scope2/2
  Sum/1 -> Sum4/2
  Constant2/1 -> Gain2/1, Gain3/1, Gain1/1, Sum3/1, Gain/1
  Gain1/1 -> Sum4/1
  Sum5/1 -> Scope4/1, Predictor (x_p_hat) dynamics/2(u)  "u"
  Gain2/1 -> Sum2/1, Sum5/1
  Sum6/1 -> [u_a]
  Gain3/1 -> Sum6/2
  Sum4/1 -> [u]
  [u] -> Sum5/2  "u"

== system UAV_Task3/Position Controller/Position controller (Kin) ==
  e_p : Inport
  Constant : Constant  Value=scenario
  Demux : Demux  Outputs=3
  If : If  IfExpression=u1 == 2
  Mux : Mux  Inputs=3
  PID Controller x : slpidlib/PID Controller  Controller=P  Form=Parallel  TimeDomain=Continuous-time  UseExternalTs=off  SampleTime=-1  IntegratorMethod=Forward Euler  FilterMethod=Forward Euler  ControllerParametersSource=internal  P=ctrl.Kpos(1,1)  I=ctrl.Kiomega(1,1)  UseKiTs=off  D=0  UseExternalDerivativeSource=off  N=100  UseFilter=on  TunerSelectOption=Transfer Function Based (PID Tuner App)  InitialConditionSource=internal  InitialConditionForIntegrator=0  InitialConditionForFilter=0  DifferentiatorICPrevScaledInput=0  ExternalReset=none  TrackingMode=off  Kt=1  LimitOutput=off  SatLimitsSource=internal  UpperSaturationLimit=inf  LowerSaturationLimit=-inf  LinearizeAsGain=on  AntiWindupMode=none  Kb=1  LimitIntegrator=off  UpperIntegratorSaturationLimit=inf  LowerIntegratorSaturationLimit=-inf  POutMin=[]  POutMax=[]  IOutMin=[]  IOutMax=[]  DOutMin=[]  DOutMax=[]  NOutMin=[]  NOutMax=[]  SumOutMin=[]  SumOutMax=[]  SaturationOutMin=[]  SaturationOutMax=[]  PParamMin=[]  PParamMax=[]  IParamMin=[]  IParamMax=[]  DParamMin=[]  DParamMax=[]  NParamMin=[]  NParamMax=[]  KbParamMin=[]  KbParamMax=[]  KtParamMin=[]  KtParamMax=[]  KbOutMin=[]  KbOutMax=[]  KtOutMin=[]  KtOutMax=[]  IntegratorOutMin=[]  IntegratorOutMax=[]  FilterOutMin=[]  FilterOutMax=[]  SumI1OutMin=[]  SumI1OutMax=[]  SumI2OutMin=[]  SumI2OutMax=[]  SumI3OutMin=[]  SumI3OutMax=[]  SumI4OutMin=[]  SumI4OutMax=[]  SumDOutMin=[]  SumDOutMax=[]  DifferentiatorOutMin=[]  DifferentiatorOutMax=[]  FilterDiffOutCoefMin=[]  FilterDiffOutCoefMax=[]  ReciprocalOutMin=[]  ReciprocalOutMax=[]  SumDenOutMin=[]  SumDenOutMax=[]  SumNumOutMin=[]  SumNumOutMax=[]  DivideOutMin=[]  DivideOutMax=[]  UdiffTsProdOutMin=[]  UdiffTsProdOutMax=[]  NTsProdOutMin=[]  NTsProdOutMax=[]  UintegralTsProdOutMin=[]  UintegralTsProdOutMax=[]  UngainTsProdOutMin=[]  UngainTsProdOutMax=[]  ClampingZeroOutDataTypeStr=Inherit: Inherit via back propagation  ClampingZeroOutMin=[]  ClampingZeroOutMax=[]  FilterDenConstantOutDataTypeStr=Inherit: Inherit via back propagation  FilterDenConstantOutMin=[]  FilterDenConstantOutMax=[]  PCopyOutDataTypeStr=Inherit: Inherit via back propagation  PCopyOutMin=[]  PCopyOutMax=[]  NCopyOutDataTypeStr=Inherit: Inherit via back propagation  NCopyOutMin=[]  NCopyOutMax=[]  IntegratorContinuousStateAttributes=''  IntegratorStateMustResolveToSignalObject=off  IntegratorRTWStateStorageClass=Auto  FilterContinuousStateAttributes=''  FilterStateMustResolveToSignalObject=off  FilterRTWStateStorageClass=Auto  ParallelPVariant=InternalParameters  IdealPVariant=Disabled  IVariant=Disabled  DVariant=Disabled  IntegratorVariant=Disabled  SatVariant=Disabled  AWVariant=Disabled  PCopyVariant=Disabled  TRVariant=Disabled  FdbkBlocksVariant=Forward  IdealPFdbkVariant=Disabled  SatFdbkVariant=Disabled  DerivativeFilterVariant=Disabled  NVariant=Disabled  NCopyVariant=Disabled_SignalSpec  FilterICVariant=Disabled  IntegratorICVariant=Disabled  ExternalResetVariant=Disabled  TRSumVariant=Passthrough  SumFdbkVariant=Disabled  SumVariant=Passthrough_P  TsampFilterVariant=InternalTs  TsampNgainVariant=Passthrough  TsampIntegralVariant=Disabled_SignalSpec  ExternalSaturationOutDataTypeStr=Inherit: Same as second input  DerivativeSourceVariant=Disabled  PreIntVariant=InternalPreInt
  PID Controller y : slpidlib/PID Controller  Controller=P  Form=Parallel  TimeDomain=Continuous-time  UseExternalTs=off  SampleTime=-1  IntegratorMethod=Forward Euler  FilterMethod=Forward Euler  ControllerParametersSource=internal  P=ctrl.Kpos(2,2)  I=ctrl.Kiomega(2,2)  UseKiTs=off  D=0  UseExternalDerivativeSource=off  N=100  UseFilter=on  TunerSelectOption=Transfer Function Based (PID Tuner App)  InitialConditionSource=internal  InitialConditionForIntegrator=0  InitialConditionForFilter=0  DifferentiatorICPrevScaledInput=0  ExternalReset=none  TrackingMode=off  Kt=1  LimitOutput=off  SatLimitsSource=internal  UpperSaturationLimit=inf  LowerSaturationLimit=-inf  LinearizeAsGain=on  AntiWindupMode=none  Kb=1  LimitIntegrator=off  UpperIntegratorSaturationLimit=inf  LowerIntegratorSaturationLimit=-inf  POutMin=[]  POutMax=[]  IOutMin=[]  IOutMax=[]  DOutMin=[]  DOutMax=[]  NOutMin=[]  NOutMax=[]  SumOutMin=[]  SumOutMax=[]  SaturationOutMin=[]  SaturationOutMax=[]  PParamMin=[]  PParamMax=[]  IParamMin=[]  IParamMax=[]  DParamMin=[]  DParamMax=[]  NParamMin=[]  NParamMax=[]  KbParamMin=[]  KbParamMax=[]  KtParamMin=[]  KtParamMax=[]  KbOutMin=[]  KbOutMax=[]  KtOutMin=[]  KtOutMax=[]  IntegratorOutMin=[]  IntegratorOutMax=[]  FilterOutMin=[]  FilterOutMax=[]  SumI1OutMin=[]  SumI1OutMax=[]  SumI2OutMin=[]  SumI2OutMax=[]  SumI3OutMin=[]  SumI3OutMax=[]  SumI4OutMin=[]  SumI4OutMax=[]  SumDOutMin=[]  SumDOutMax=[]  DifferentiatorOutMin=[]  DifferentiatorOutMax=[]  FilterDiffOutCoefMin=[]  FilterDiffOutCoefMax=[]  ReciprocalOutMin=[]  ReciprocalOutMax=[]  SumDenOutMin=[]  SumDenOutMax=[]  SumNumOutMin=[]  SumNumOutMax=[]  DivideOutMin=[]  DivideOutMax=[]  UdiffTsProdOutMin=[]  UdiffTsProdOutMax=[]  NTsProdOutMin=[]  NTsProdOutMax=[]  UintegralTsProdOutMin=[]  UintegralTsProdOutMax=[]  UngainTsProdOutMin=[]  UngainTsProdOutMax=[]  ClampingZeroOutDataTypeStr=Inherit: Inherit via back propagation  ClampingZeroOutMin=[]  ClampingZeroOutMax=[]  FilterDenConstantOutDataTypeStr=Inherit: Inherit via back propagation  FilterDenConstantOutMin=[]  FilterDenConstantOutMax=[]  PCopyOutDataTypeStr=Inherit: Inherit via back propagation  PCopyOutMin=[]  PCopyOutMax=[]  NCopyOutDataTypeStr=Inherit: Inherit via back propagation  NCopyOutMin=[]  NCopyOutMax=[]  IntegratorContinuousStateAttributes=''  IntegratorStateMustResolveToSignalObject=off  IntegratorRTWStateStorageClass=Auto  FilterContinuousStateAttributes=''  FilterStateMustResolveToSignalObject=off  FilterRTWStateStorageClass=Auto  ParallelPVariant=InternalParameters  IdealPVariant=Disabled  IVariant=Disabled  DVariant=Disabled  IntegratorVariant=Disabled  SatVariant=Disabled  AWVariant=Disabled  PCopyVariant=Disabled  TRVariant=Disabled  FdbkBlocksVariant=Forward  IdealPFdbkVariant=Disabled  SatFdbkVariant=Disabled  DerivativeFilterVariant=Disabled  NVariant=Disabled  NCopyVariant=Disabled_SignalSpec  FilterICVariant=Disabled  IntegratorICVariant=Disabled  ExternalResetVariant=Disabled  TRSumVariant=Passthrough  SumFdbkVariant=Disabled  SumVariant=Passthrough_P  TsampFilterVariant=InternalTs  TsampNgainVariant=Passthrough  TsampIntegralVariant=Disabled_SignalSpec  ExternalSaturationOutDataTypeStr=Inherit: Same as second input  DerivativeSourceVariant=Disabled  PreIntVariant=InternalPreInt
  PID Controller z : slpidlib/PID Controller  Controller=P  Form=Parallel  TimeDomain=Continuous-time  UseExternalTs=off  SampleTime=-1  IntegratorMethod=Forward Euler  FilterMethod=Forward Euler  ControllerParametersSource=internal  P=ctrl.Kpos(3,3)  I=ctrl.Kiomega(3,3)  UseKiTs=off  D=0  UseExternalDerivativeSource=off  N=100  UseFilter=on  TunerSelectOption=Transfer Function Based (PID Tuner App)  InitialConditionSource=internal  InitialConditionForIntegrator=0  InitialConditionForFilter=0  DifferentiatorICPrevScaledInput=0  ExternalReset=none  TrackingMode=off  Kt=1  LimitOutput=off  SatLimitsSource=internal  UpperSaturationLimit=inf  LowerSaturationLimit=-inf  LinearizeAsGain=on  AntiWindupMode=none  Kb=1  LimitIntegrator=off  UpperIntegratorSaturationLimit=inf  LowerIntegratorSaturationLimit=-inf  POutMin=[]  POutMax=[]  IOutMin=[]  IOutMax=[]  DOutMin=[]  DOutMax=[]  NOutMin=[]  NOutMax=[]  SumOutMin=[]  SumOutMax=[]  SaturationOutMin=[]  SaturationOutMax=[]  PParamMin=[]  PParamMax=[]  IParamMin=[]  IParamMax=[]  DParamMin=[]  DParamMax=[]  NParamMin=[]  NParamMax=[]  KbParamMin=[]  KbParamMax=[]  KtParamMin=[]  KtParamMax=[]  KbOutMin=[]  KbOutMax=[]  KtOutMin=[]  KtOutMax=[]  IntegratorOutMin=[]  IntegratorOutMax=[]  FilterOutMin=[]  FilterOutMax=[]  SumI1OutMin=[]  SumI1OutMax=[]  SumI2OutMin=[]  SumI2OutMax=[]  SumI3OutMin=[]  SumI3OutMax=[]  SumI4OutMin=[]  SumI4OutMax=[]  SumDOutMin=[]  SumDOutMax=[]  DifferentiatorOutMin=[]  DifferentiatorOutMax=[]  FilterDiffOutCoefMin=[]  FilterDiffOutCoefMax=[]  ReciprocalOutMin=[]  ReciprocalOutMax=[]  SumDenOutMin=[]  SumDenOutMax=[]  SumNumOutMin=[]  SumNumOutMax=[]  DivideOutMin=[]  DivideOutMax=[]  UdiffTsProdOutMin=[]  UdiffTsProdOutMax=[]  NTsProdOutMin=[]  NTsProdOutMax=[]  UintegralTsProdOutMin=[]  UintegralTsProdOutMax=[]  UngainTsProdOutMin=[]  UngainTsProdOutMax=[]  ClampingZeroOutDataTypeStr=Inherit: Inherit via back propagation  ClampingZeroOutMin=[]  ClampingZeroOutMax=[]  FilterDenConstantOutDataTypeStr=Inherit: Inherit via back propagation  FilterDenConstantOutMin=[]  FilterDenConstantOutMax=[]  PCopyOutDataTypeStr=Inherit: Inherit via back propagation  PCopyOutMin=[]  PCopyOutMax=[]  NCopyOutDataTypeStr=Inherit: Inherit via back propagation  NCopyOutMin=[]  NCopyOutMax=[]  IntegratorContinuousStateAttributes=''  IntegratorStateMustResolveToSignalObject=off  IntegratorRTWStateStorageClass=Auto  FilterContinuousStateAttributes=''  FilterStateMustResolveToSignalObject=off  FilterRTWStateStorageClass=Auto  ParallelPVariant=InternalParameters  IdealPVariant=Disabled  IVariant=Disabled  DVariant=Disabled  IntegratorVariant=Disabled  SatVariant=Disabled  AWVariant=Disabled  PCopyVariant=Disabled  TRVariant=Disabled  FdbkBlocksVariant=Forward  IdealPFdbkVariant=Disabled  SatFdbkVariant=Disabled  DerivativeFilterVariant=Disabled  NVariant=Disabled  NCopyVariant=Disabled_SignalSpec  FilterICVariant=Disabled  IntegratorICVariant=Disabled  ExternalResetVariant=Disabled  TRSumVariant=Passthrough  SumFdbkVariant=Disabled  SumVariant=Passthrough_P  TsampFilterVariant=InternalTs  TsampNgainVariant=Passthrough  TsampIntegralVariant=Disabled_SignalSpec  ExternalSaturationOutDataTypeStr=Inherit: Same as second input  DerivativeSourceVariant=Disabled  PreIntVariant=InternalPreInt
  Subsystem : Subsystem
  Terminator : Terminator
  v_c : Outport
  wires:
  PID Controller y/1 -> Mux/2
  Demux/2 -> PID Controller y/1
  e_p/1 -> Demux/1, Subsystem/1(e_p)
  Demux/3 -> PID Controller z/1
  PID Controller x/1 -> Mux/1
  PID Controller z/1 -> Mux/3
  Demux/1 -> PID Controller x/1
  Mux/1 -> v_c/1
  Constant/1 -> If/1
  If/1 -> Subsystem/Action
  If/2 -> Terminator/1

== system UAV_Task3/Position Controller/Sat ==
  In1 : Inport
  Demux : Demux  Outputs=3
  Mux : Mux  Inputs=3
  Saturation : Saturate  UpperLimit=0  LowerLimit=-1000
  Scope : Scope
  Scope1 : Scope  NumInputPorts=2
  Out1 : Outport
  wires:
  Mux/1 -> Scope/1, Out1/1
  In1/1 -> Demux/1
  Demux/1 -> Mux/1
  Demux/2 -> Mux/2
  Demux/3 -> Scope1/2, Saturation/1
  Saturation/1 -> Scope1/1, Mux/3

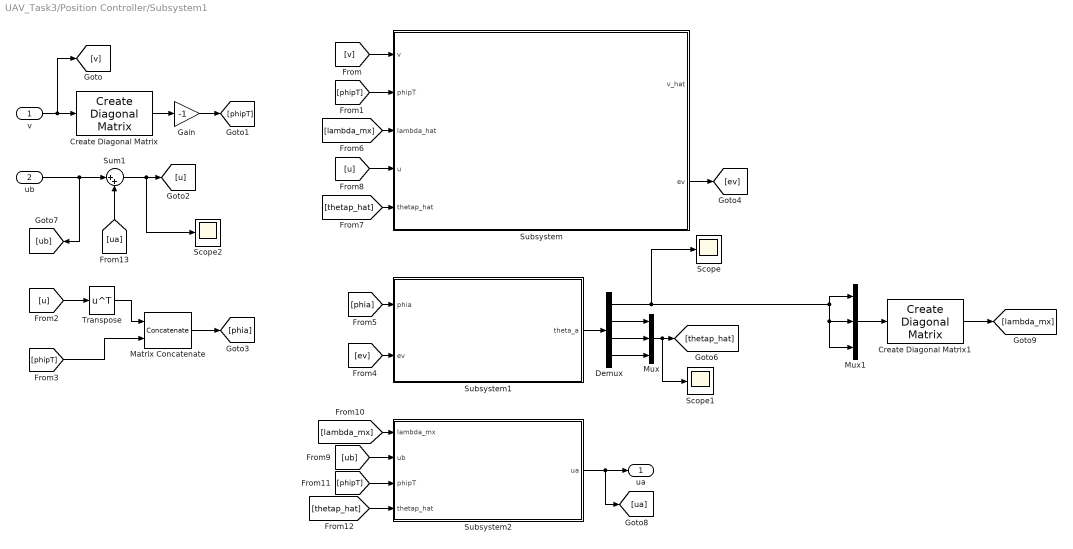
== system UAV_Task3/Position Controller/Subsystem1 ==
  v : Inport
  ub : Inport  Port=2
  Create Diagonal Matrix : matrix_library/Create Diagonal Matrix
  Create Diagonal Matrix1 : matrix_library/Create Diagonal Matrix
  Demux : Demux
  Gain : Gain  Gain=-1
  Matrix Concatenate : Concatenate  Mode=Multidimensional array
  Mux : Mux  Inputs=3
  Mux1 : Mux  Inputs=3
  Scope : Scope
  Scope1 : Scope
  Scope2 : Scope
  Subsystem : Subsystem
  Subsystem1 : Subsystem
  Subsystem2 : Subsystem
  Sum1 : Sum  Inputs=|++
  Transpose : Math  Operator=transpose
  ua : Outport
  wires:
  v/1 -> [v], Create Diagonal Matrix/1
  ub/1 -> Sum1/1, [ub]
  [v] -> Subsystem/1(v)
  [phipT] -> Subsystem/2(phipT)
  [phipT] -> Matrix Concatenate/2
  Subsystem/2(ev) -> [ev]
  [ev] -> Subsystem1/2(ev)
  [phia] -> Subsystem1/1(phia)
  Subsystem1/1(theta_a) -> Demux/1
  Demux/4 -> Mux/3
  Demux/3 -> Mux/2
  Demux/2 -> Mux/1
  Mux/1 -> Scope1/1, [thetap_hat]
  [lambda_mx] -> Subsystem/3(lambda_hat)
  [thetap_hat] -> Subsystem/5(thetap_hat)
  [u] -> Subsystem/4(u)
  [ub] -> Subsystem2/2(ub)
  [phipT] -> Subsystem2/3(phipT)
  [thetap_hat] -> Subsystem2/4(thetap_hat)
  Subsystem2/1(ua) -> [ua], ua/1
  [ua] -> Sum1/2
  Demux/1 -> Scope/1, Mux1/1, Mux1/3, Mux1/2
  Mux1/1 -> Create Diagonal Matrix1/1
  Create Diagonal Matrix1/1 -> [lambda_mx]
  [lambda_mx] -> Subsystem2/1(lambda_mx)
  Create Diagonal Matrix/1 -> Gain/1
  Gain/1 -> [phipT]
  [u] -> Transpose/1
  Matrix Concatenate/1 -> [phia]
  Sum1/1 -> Scope2/1, [u]
  Transpose/1 -> Matrix Concatenate/1
